simulink model "MultirotorSimPx4HorThrust"  (R2020b)
settings: Solver=VariableStepAuto  StartTime=0.0  StopTime=Simulation.T_END  MaxStep=Simulation.TS_MAX  RelTol=1e-3  EnableMultiTasking=on
PreLoadFcn:
  | % InitializeParameters;
undefined symbols (not defined in the file): Initial, Simulation, Uav
libraries: QuaternionLibrary x26, Px4Library x7, simulink_extras x3
(part 1 of 2)
settings Model: PauseTimes=30  Creator=jban039  LastModifiedBy=jban039
settings DataIOCC: Decimation=10  InitialState=getstatestruct(op)  SaveFormat=StructureWithTime  OutputTimes=Simulation.T_OUT
settings OptimizationCC: LifeSpan=inf
settings DebuggingCC: ReadBeforeWriteMsg=DisableAll  WriteAfterWriteMsg=DisableAll  WriteAfterReadMsg=DisableAll  MultiTaskDSMMsg=none  UnconnectedLineMsg=none  AllowSymbolicDim=off  SFUnexpectedBacktrackingDiag=warning  SFNoUnconditionalDefaultTransitionDiag=warning  SFExecutionAtInitializationDiag=none  ArithmeticOperatorsInVariantConditions=warning
settings ModelReferenceCC: UpdateModelReferenceTargets=IfOutOfDate  ModelReferenceMinAlgLoopOccurrences=on  PropagateSignalLabelsOutOfModel=off
settings SFSimCC: SFSimEcho=off  SimUseLocalCustomCode=off  CustomCodeUndefinedFunction=UseInterfaceOnly
settings RTWCC: RTWUseLocalCustomCode=off
settings CodeAppCC: StateflowObjectComments=on
settings GRTTargetCC: TargetLangStandard=C89/C90 (ANSI)
settings ConfigComp: CovMetricSettings=dw  CovSaveCumulativeToWorkspaceVar=on  CovSaveSingleToWorkspaceVar=on  CovExternalEMLEnable=off

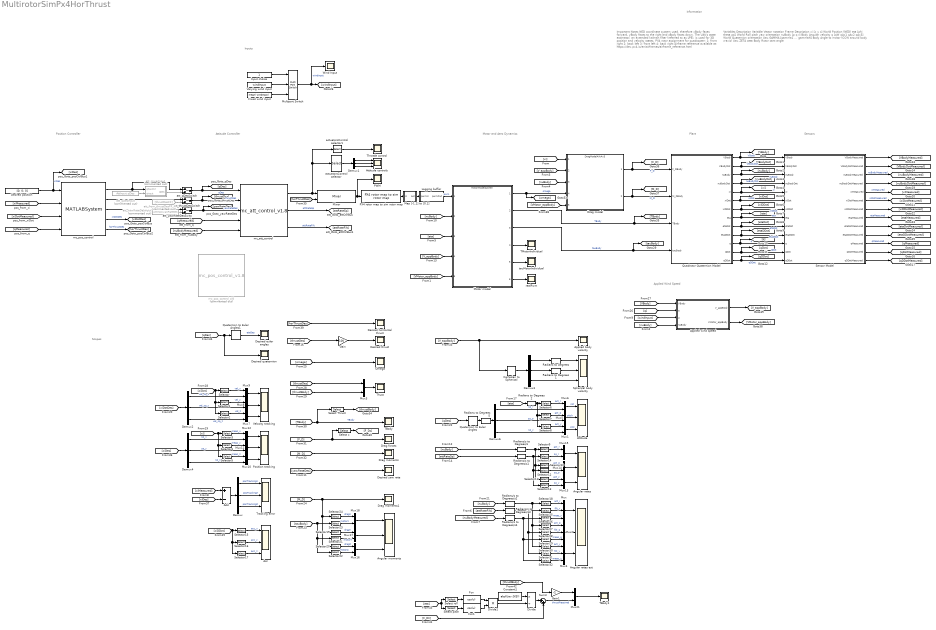
== system MultirotorSimPx4HorThrust ==
  note: Important Notes
      |
      | NED coordinate system used, therefore xBody faces forward, yBody faces to the right and zBody faces down.
      | The UAV's state estimator, an extended kalman filter (referred to as LPE), is used for 3D position and velocity states.
      | PX4 rotor assignment for quadcopter:
      | 1: front right
      | 2: back left
      | 3: front left
      | 4: back right
      | Airframe reference available at:
      | https://dev.px4.io/en/airframes/airframe_reference.html
  note: Applied Wind Speed
  note: Inputs
  note: Scopes
  note: Information
  note: Plant
  note: Motor and Aero Dynamics
  note: Sensors
  note: Attitude Controller
  note: Position Controller
  note: Variables Description
      |
      | Variable
      | Vector notation
      | Frame
      | Description
      |
      | xi
      | [x y z]
      | World
      | Position (NED)
      |
      | eta
      | [phi theta psi]
      | World
      | Roll pitch yaw orientation
      |
      | nuBody
      | [p q r]
      | Body
      | Angular velocity
      |
      | q
      | [qW qAx1 qAx2 qAx3]
      | World
      | Quaternion orientation
      |
      | Uav.GAMMA
      | [gamma1 ... gammaN]
      | Body
      | Angle to motor (CCW around body z-axis)
      |
      | Uav.ZETA
      | zeta
      | Body
      | Rotor cant angle
  Acc : Scope  NumInputPorts=3
  Add : Sum  Inputs=+-
  Angular moments : Scope  NumInputPorts=3
  Angular rates : Scope  NumInputPorts=3
  Angular rates est : Scope  NumInputPorts=3
  Applied body velocity : Scope
  Applied wind speed : Subsystem
  Attitude : Scope  NumInputPorts=3
  Attitude controls : Scope  NumInputPorts=3
  Cartesian to Spherical : QuaternionLibrary/Cartesian to Spherical
  Constant1 : Constant  Value=abs(Uav.G(3))
  Demux{,1..4,6} (6 alike) : Demux  Outputs=3
  Desired euler angles : Scope
  Desired horizontal thrust : Scope
  Desired quaternion : Scope
  Desired thrust : Scope
  Desired position : Constant  Value=[0; 0; 0]
  Desired yaw rate : Scope
  Divide : Product  Inputs=*/
  Divide1 : Product  Inputs=**
  Drag forces : Scope
  Drag model : ModelReference  ModelNameDialog=DragModelAIAAv3  SimulationMode=Normal  ModelReferenceVersion=5.2
  Drag moments : Scope
  Drag moments1 : Scope
  Fcn : Fcn  Expr=cos(u)
  Fcn1 : Fcn  Expr=cos(u)
  Fixed wind input : Constant  Value=mean( windInput )
  Gain : Gain  Gain=100
  Gain1 : Gain  Gain=-1
  Input choice : Constant
  Logging buffer : Subsystem
  Map [-1,1] to [0,1] : Subsystem
  Mixer : Px4Library/Mixer  airframeConfig=5  useHorThrust=1  outputSatStatus=0  SimulateUsing=Code generation
  Motor model : ModelReference  ModelNameDialog=MotorModelZJChen  SimulationMode=Normal  ModelReferenceVersion=5.15
  Multiport Switch : MultiPortSwitch  Inputs=2
  Mux : Mux  Inputs=3
  Mux{1,3,5..18,21} (17 alike) : Mux  Inputs=2
  Mux2 : Mux  Inputs=3
  Mux4 : Mux  Inputs=3
  Omega : Scope
  PWM : Scope
  PX4 rotor map to sim rotor map : Px4Library/PX4 rotor map to sim rotor map  airframeConfig=5  SimulateUsing=Code generation
  Position tracking : Scope  NumInputPorts=3
  Quadrotor Quaternion Model : Subsystem
  Quaternion to Euler Angles : QuaternionLibrary/Quaternion to Euler Angles
  Quaternion to Euler Angles1 : QuaternionLibrary/Quaternion to Euler Angles
  Radians to Degrees {,1..2,5} (4 alike) : QuaternionLibrary/Radians to Degrees   SystemSampleTime=-1  VariantActivationTime=update diagram  Latency=0  AutoFrameSizeCalculation=off
  Radians/s to Degrees/s{,1..4} (5 alike) : QuaternionLibrary/Radians//s to Degrees//s  SystemSampleTime=-1  VariantActivationTime=update diagram  Latency=0  AutoFrameSizeCalculation=off
  Select Thrust : Selector  InputPortWidth=3  IndexOptions=Index vector (dialog)  Indices=[3]  OutputSizes=1
  Select pitch : Selector  InputPortWidth=3  IndexOptions=Index vector (dialog)  Indices=2  OutputSizes=1
  Select roll : Selector  InputPortWidth=3  IndexOptions=Index vector (dialog)  Indices=1  OutputSizes=1
  Select z : Selector  InputPortWidth=3  IndexOptions=Index vector (dialog)  Indices=[3]  OutputSizes=1
  Selector{,3,6,9,14..15,18,23..26} (11 alike) : Selector  InputPortWidth=3  IndexOptions=Index vector (dialog)  Indices=1  OutputSizes=1
  Selector{1,4,7,10,12,16,19,21,27..29} (11 alike) : Selector  InputPortWidth=3  IndexOptions=Index vector (dialog)  Indices=2  OutputSizes=1
  Selector{2,5,8,11,13,17,20,22,30..32} (11 alike) : Selector  InputPortWidth=3  IndexOptions=Index vector (dialog)  Indices=3  OutputSizes=1
  Sensor Model : Subsystem
  Spherical body velocity : Scope  NumInputPorts=3
  Sum3 : Sum  Inputs=|++
  TBody : Scope
  TBody1 : Scope
  TMotorIndividual : Scope
  Throttle control : Scope
  Thust : Scope
  Tracking error : Scope  NumInputPorts=3
  Varying wind input : FromWorkspace  VariableName=windInput
  Velocity tracking : Scope  NumInputPorts=3
  Wind Input : Scope
  actuatorsControl selector : Selector  InputPortWidth=8  IndexOptions=Index vector (dialog)  Indices=[1 2 3]  OutputSizes=1
  actuatorsControl selector1 : Selector  InputPortWidth=8  IndexOptions=Index vector (dialog)  Indices=4  OutputSizes=1
  att_from_thrustDesFF_ff : From  Commented=on  GotoTag=thrustDesFF
  att_mixerInput : Subsystem  Commented=on
  att_qDesInput : FromWorkspace  Commented=on  VariableName=AttInput.qDes  Interpolate=off  OutputAfterFinalValue=Holding final value
  att_qDesSwitch : ManualSwitch
  att_thrustDesSwitch : ManualSwitch
  att_yawRateDesInput : FromWorkspace  Commented=on  VariableName=AttInput.yawRateDes  Interpolate=off  OutputAfterFinalValue=Holding final value
  att_yawRateDesSwitch : ManualSwitch
  mc_att_control : Px4Library/mc_att_control_v1.8  acro_expo_rp=0.69  acro_expo_y=0.69  acro_pitch_max=720  acro_roll_max=720  acro_superexpo_rp=0.7  acro_superexpo_y=0.7  acro_yaw_max=540  airmode=0  d_term_cutoff_freq=30  pitch_rate_d=0.003  pitch_rate_ff=0  pitch_rate_i=0.05  pitch_rate_max=220  pitch_rate_p=0.15  pitch_p=6.5  pitch_rate_integ_lim=0.3  rattitude_thres=0.8  roll_rate_d=0.003  roll_rate_ff=0  roll_rate_i=0.05  roll_rate_max=220  roll_rate_p=0.15  roll_p=6.5  roll_rate_integ_lim=0.3  tpa_breakpoint_d=1  tpa_breakpoint_i=1  tpa_breakpoint_p=1  tpa_rate_d=0  tpa_rate_i=0  tpa_rate_p=0  yaw_rate_d=0  yaw_rate_ff=0  yaw_rate_i=0.1  yaw_rate_max=200  yaw_rate_p=0.2  yaw_auto_max=45  yaw_p=2.8  yaw_rate_integ_lim=0.3  man_throttle_min=0.08  man_tilt_max_deg=35  yaw_rate_scaling=200  throttle_hover=0.5370  throttle_max=1  board_rotation_param=0  board_offset_x=0  board_offset_y=0  board_offset_z=0  bat_scale_en=0  throttle_curve=0  vehicle_status_is_rotary_wing=1  vehicle_status_is_vtol=0  loop_update_rate_hz=250  simple_mode=1  output_rates=1  SimulateUsing=Code generation
  mc_pos_control : MATLABSystem  System=MulticopterPositionControlHorizontal  global_yaw_max_deg=200  mc_att_yaw_p=2.8  mis_yaw_error=12  acceleration_z_max_down=10  acceleration_hor=5  acc_max_estimator_xy=0.5  acceleration_hor_max=10  acceleration_z_max_up=10  alt_mode=0  cruise_speed_90=3  deceleration_hor_slow=5  test_flight_tasks=0  hold_dz=0.1  hold_max_xy=0.8  hold_max_z=0.6  jerk_hor_max=0  jerk_hor_min=1  slow_land_alt1=10  slow_land_alt2=5  land_speed=0.7  manual_thr_max=1  manual_thr_min=0.08  man_tilt_max_deg=35  man_yaw_max_deg=200  thr_hover=0.5  thr_max=1  thr_min=0.12  tilt_max_air_deg=45  tilt_max_land_deg=12  takeoff_ramp_time=0.4  tko_speed=1.5  veld_lp=5  velocity_hor_manual=10  vel_cruise_xy=5  xy_vel_man_expo=0  xy_p=0.95  xy_vel_d=0.01  xy_vel_i=0.02  vel_max_xy_param=12  xy_vel_p=0.09  z_vel_man_expo=0  z_p=1  z_vel_d=0  z_vel_i=0.02  vel_max_down=1  vel_max_up=3  z_vel_p=0.2  nav_rad=10  rc_flt_cutoff=10  rc_flt_smp_rate=50  loop_update_rate_hz=50  simple_mode=1  start_landed=0  ref_lat_init=-36.8509  ref_lon_init=174.7645  ref_alt_init=19  use_hor_thrust=1  controller=Ctrl  controller_op=thrustOp  SimulateUsing=Code generation
      mask Type: MulticopterPositionControlHorizontal
      mask Display:
      | disp(['mc_pos_control' char(10) '' char(10) 'v1.82' char(10) '' char(10) 'HORIZONTAL']);
      | port_label('input',1,'xiDes');
      | port_label('input',2,'xiMeas');
      | port_label('input',3,'xiDotMeas');
      | port_label('input',4,'qMeas');
      | port_label('output',1,'qDes');
      | port_label('output',2,'thrustDes');
      | port_label('output',3,'yawRateDes');
      | port_label('output',4,'xiDotDes');
      | port_label('output',5,'horThrustDes');
  mc_pos_control_old : Px4Library/mc_pos_control_v1.8  Commented=on  global_yaw_max_deg=200  mc_att_yaw_p=2.8  mis_yaw_error=12  acceleration_z_max_down=10  acceleration_hor=5  acc_max_estimator_xy=0.5  acceleration_hor_max=10  acceleration_z_max_up=10  alt_mode=0  cruise_speed_90=3  deceleration_hor_slow=5  test_flight_tasks=0  hold_dz=0.1  hold_max_xy=0.8  hold_max_z=0.6  jerk_hor_max=0  jerk_hor_min=1  slow_land_alt1=1  slow_land_alt2=0.5  land_speed=0.6  manual_thr_max=1  manual_thr_min=0.08  man_tilt_max_deg=35  man_yaw_max_deg=200  thr_hover=0.5370  thr_max=1  thr_min=0.12  tilt_max_air_deg=45  tilt_max_land_deg=12  takeoff_ramp_time=0.4  tko_speed=1.5  veld_lp=5  velocity_hor_manual=10  vel_cruise_xy=5  xy_vel_man_expo=0  xy_p=0.95  xy_vel_d=0.01  xy_vel_i=0.02  vel_max_xy_param=12  xy_vel_p=0.09  z_vel_man_expo=0  z_p=1  z_vel_d=0  z_vel_i=0.02  vel_max_down=1  vel_max_up=3  z_vel_p=0.2  nav_rad=2  rc_flt_cutoff=10  rc_flt_smp_rate=50  loop_update_rate_hz=50  simple_mode=1  start_landed=0  ref_lat_init=-36.8509  ref_lon_init=174.7645  ref_alt_init=19  SimulateUsing=Code generation
  realPwm : Scope
  tauMotorIndividual : Scope
  wires:
  Motor model/1 -> [omega], Drag model/4  "omega"
  Motor model/2 -> Quadrotor Quaternion Model/3(TBody), [TBody]  "TBody"
  Drag model/2 -> Quadrotor Quaternion Model/2(M_DBody), [M_D]  "M_D"
  Quadrotor Quaternion Model/1(VBody) -> Sensor Model/1(VBody), [VBody]  "VBody"
  Quadrotor Quaternion Model/2(VBodyDot) -> Sensor Model/2(VBodyDot), [VBodyDot]  "VBodyDot"
  Quadrotor Quaternion Model/3(nuBody) -> Sensor Model/3(nuBody), [nuBody]  "nuBody"
  Quadrotor Quaternion Model/4(nuBodyDot) -> Sensor Model/4(nuBodyDot), [nuBodyDot]  "nuBodyDot"
  Quadrotor Quaternion Model/5(xi) -> Sensor Model/5(xi), [xi]  "xi"
  Quadrotor Quaternion Model/6(xiDot) -> Sensor Model/6(xiDot), [xiDot]  "xiDot"
  Quadrotor Quaternion Model/7(xiDDot) -> Sensor Model/7(xiDDot), [xiDDot]  "xiDDot"
  Quadrotor Quaternion Model/8(eta) -> Sensor Model/8(eta), [eta]  "eta"
  Quadrotor Quaternion Model/9(etaDot) -> Sensor Model/9(etaDot), [etaDot]  "etaDot"
  Quadrotor Quaternion Model/10(etaDDot) -> Sensor Model/10(etaDDot), [etaDDot]  "etaDDot"
  [V_appBody] -> Drag model/2
  [nuBody] -> Motor model/2
  Quadrotor Quaternion Model/11(q) -> Sensor Model/11(q), [q]  "q"
  Quadrotor Quaternion Model/12(qDot) -> Sensor Model/12(qDot), [qDot]  "qDot"
  Quadrotor Quaternion Model/13(qDDot) -> Sensor Model/13(qDDot), [qDDot]  "qDDot"
  Drag model/1 -> Quadrotor Quaternion Model/1(F_DBody), [F_D]  "F_D"
  Sensor Model/1(VBodyMeasured) -> [VBodyMeasured]
  Sensor Model/2(VBodyDotMeasured) -> [VBodyDotMeasured]
  Sensor Model/3(nuBodyMeasured) -> [nuBodyMeasured]  "nuBodyMeasured"
  Sensor Model/4(nuBodyDotMeasured) -> [nuBodyDotMeasured]
  Sensor Model/5(xiMeasured) -> [xiMeasured]  "xiMeasured"
  Sensor Model/6(xiDotMeasured) -> [xiDotMeasured]  "xiDotMeasured"
  Sensor Model/7(xiDDotMeasured) -> [xiDDotMeasured]
  Sensor Model/8(etaMeasured) -> [etaMeasured]  "etaMeasured"
  Sensor Model/9(etaDotMeasured) -> [etaDotMeasured]
  Sensor Model/10(etaDDotMeasured) -> [etaDDotMeasured]
  Sensor Model/11(qMeasured) -> [qMeasured]  "qMeasured"
  Sensor Model/12(qDotMeasured) -> [qDotMeasured]
  Sensor Model/13(qDDotMeasured) -> [qDDotMeasured]
  Logging buffer/1(pwmOut) -> Motor model/1  "pwm"
  [qMeasured] -> mc_att_control/4
  [nuBodyMeasured] -> mc_att_control/5
  [qMeasured] -> mc_pos_control/4
  mc_pos_control/3 -> att_yawRateDesSwitch/1
  [xiDotMeasured] -> mc_pos_control/3
  [xiMeasured] -> mc_pos_control/2
  Selector6/1 -> Mux6/1  "act_r"
  Selector7/1 -> Mux5/1  "act_p"
  Mux7/1 -> Velocity tracking/3
  Mux8/1 -> Velocity tracking/2
  Mux9/1 -> Velocity tracking/1
  Demux2/1 -> Mux9/2  "vel_sp_x"
  Selector/1 -> Mux9/1  "vel_x"
  Demux2/2 -> Mux8/2  "vel_sp_y"
  Selector1/1 -> Mux8/1  "vel_y"
  Demux2/3 -> Mux7/2  "vel_sp_z"
  Selector2/1 -> Mux7/1  "vel_z"
  Mux10/1 -> Position tracking/3
  Mux11/1 -> Position tracking/2
  Mux12/1 -> Position tracking/1
  Demux4/1 -> Mux12/2  "sp_x"
  Selector3/1 -> Mux12/1  "meas_x"
  Demux4/2 -> Mux11/2  "sp_y"
  Selector4/1 -> Mux11/1  "meas_y"
  Demux4/3 -> Mux10/2  "sp_z"
  Selector5/1 -> Mux10/1  "meas_z"
  Quaternion to Euler Angles/1 -> Radians to Degrees 5/1
  Demux6/1 -> Mux6/2  "sp_r"
  Demux6/2 -> Mux5/2  "sp_p"
  Demux6/3 -> Mux1/2  "sp_y"
  Selector8/1 -> Mux1/1  "act_y"
  [qDes] -> Quaternion to Euler Angles/1
  Mixer/1 -> PX4 rotor map to sim rotor map/1, PWM/1
  Map [-1,1] to [0,1]/1(out) -> Logging buffer/1(pwmIn)
  Add/1 -> Demux/1
  Demux/1 -> Tracking error/1  "posTrackingX"
  Demux/2 -> Tracking error/2  "posTrackingY"
  Demux/3 -> Tracking error/3  "posTrackingZ"
  [nuBody] -> Drag model/3
  Mux6/1 -> Attitude/1  "roll"
  Mux5/1 -> Attitude/2  "pitch"
  [eta] -> Motor model/3
  [xiDot] -> Selector2/1, Selector1/1, Selector/1
  [xi] -> Selector5/1, Selector4/1, Selector3/1
  [xiMeasured] -> Add/1
  Multiport Switch/1 -> Wind Input/1, [windInput]  "windInput"
  [V_appBody] -> Motor model/4
  mc_pos_control/4 -> [xiDotDes]  "xiDotDes"
  mc_att_control/2 -> [attRateSp]  "attRateSp"
  [omega] -> Omega/1
  Radians to Degrees 5/1 -> Demux6/1
  Radians to Degrees 2/1 -> Selector8/1, Selector7/1, Selector6/1
  [eta] -> Radians to Degrees 2/1
  Motor model/4 -> TMotorIndividual/1
  [thrustDes] -> Mux3/1
  [thrustBody] -> Mux3/2
  Mux3/1 -> Thust/1
  Motor model/5 -> tauMotorIndividual/1
  [xi] -> Drag model/1
  [TBody] -> Select Thrust/1, TBody/1  "TBody"
  Select Thrust/1 -> [thrustBody]
  [F_D] -> Drag forces/1, Select z/1
  [V_appBody] -> Cartesian to Spherical/1, Applied body velocity/1
  Demux3/1 -> "Radians to Degrees "/1
  Demux3/2 -> Radians to Degrees 1/1
  Demux3/3 -> Spherical body velocity/3
  "Radians to Degrees "/1 -> Spherical body velocity/1
  Radians to Degrees 1/1 -> Spherical body velocity/2
  [M_D] -> Drag moments/1
  [VMotor_appBody] -> Motor model/5
  [VMotor_appBody] -> Drag model/5
  att_qDesSwitch/1 -> mc_att_control/1, [qDes]  "qDes"
  att_thrustDesSwitch/1 -> mc_att_control/2, [thrustDes]  "thrustDes"
  att_yawRateDesSwitch/1 -> mc_att_control/3, [yawRateDes]  "yawRateDes"
  att_yawRateDesInput/1 -> att_yawRateDesSwitch/2
  att_from_thrustDesFF_ff/1 -> att_thrustDesSwitch/2
  [yawRateDes] -> Desired yaw rate/1
  Mux1/1 -> Attitude/3  "yaw"
  Motor model/3 -> Quadrotor Quaternion Model/4(tauBody), [tauBody]  "tauBody"
  [VBody] -> Applied wind speed/1(VBody)
  [q] -> Applied wind speed/2(q)
  [windInput] -> Applied wind speed/3(U)
  Applied wind speed/1(V_appBody) -> [V_appBody]
  Applied wind speed/2(VMotor_appBody) -> [VMotor_appBody]
  [nuBody] -> Applied wind speed/4(nuBody)
  Selector9/1 -> Mux15/1  "act_r"
  Selector10/1 -> Mux14/1  "act_p"
  Selector11/1 -> Mux13/1  "act_y"
  Mux15/1 -> Angular rates/1
  Mux14/1 -> Angular rates/2
  Radians/s to Degrees/s/1 -> Selector9/1, Selector11/1, Selector10/1
  [nuBody] -> Radians/s to Degrees/s/1
  Mux13/1 -> Angular rates/3
  Radians/s to Degrees/s1/1 -> Selector14/1, Selector13/1, Selector12/1
  Selector14/1 -> Mux15/2  "sp_r"
  Selector12/1 -> Mux14/2  "sp_p"
  Selector13/1 -> Mux13/2  "sp_y"
  [attRateSp] -> Radians/s to Degrees/s1/1
  Selector15/1 -> Acc/1  "acc_x"
  Selector16/1 -> Acc/2  "acc_y"
  Selector17/1 -> Acc/3  "acc_z"
  [xiDDot] -> Selector15/1, Selector16/1, Selector17/1
  [thrustDes] -> Gain/1
  actuatorsControl selector/1 -> Demux1/1
  [M_D] -> Selector20/1, Selector19/1, Selector24/1, Drag moments1/1
  Mux18/1 -> Angular moments/1
  Mux17/1 -> Angular moments/2
  Mux16/1 -> Angular moments/3
  Selector24/1 -> Mux18/1  "dragX"
  Selector23/1 -> Mux18/2  "motorX"
  Selector19/1 -> Mux17/1  "dragY"
  Selector21/1 -> Mux17/2  "motorY"
  Selector20/1 -> Mux16/1  "dragZ"
  Selector22/1 -> Mux16/2  "MotorZ"
  [tauBody] -> Selector22/1, Selector21/1, Selector23/1
  Desired position/1 -> [xiDes], mc_pos_control/1  "xiDes"
  [qDes] -> Desired quaternion/1, Quaternion to Euler Angles1/1
  Quaternion to Euler Angles1/1 -> Desired euler angles/1  "etaDes"
  Divide/1 -> Sum3/1
  Sum3/1 -> Mux21/2  "thrustRequired"
  Mux21/1 -> TBody1/1
  Constant1/1 -> Divide/1
  Select z/1 -> [F_Dz]
  [thrustBody] -> Gain1/1
  [eta] -> Select pitch/1, Select roll/1
  Select roll/1 -> Fcn/1
  Select pitch/1 -> Fcn1/1
  Fcn/1 -> Divide1/1
  Fcn1/1 -> Divide1/2
  Divide1/1 -> Divide/2
  [F_Dz] -> Sum3/2
  mc_pos_control/1 -> att_qDesSwitch/1, att_mixerInput/1(qPosCtrl)
  mc_pos_control/2 -> att_thrustDesSwitch/1
  att_mixerInput/1(qDes) -> att_qDesSwitch/2
  att_qDesInput/1 -> att_mixerInput/2(qInput)
  Motor model/6 -> realPwm/1
  Cartesian to Spherical/1 -> Demux3/1
  mc_att_control/1 -> actuatorsControl selector1/1, actuatorsControl selector/1, Mixer/1
  Input choice/1 -> Multiport Switch/1
  Fixed wind input/1 -> Multiport Switch/3
  Varying wind input/1 -> Multiport Switch/2
  [xiDotDes] -> Demux2/1
  [xiDes] -> Demux4/1
  [xiDes] -> Add/2
  Gain/1 -> Desired thrust/1
  mc_att_control/3 -> [attRateFilt]  "attRateFilt"
  [nuBody] -> Radians/s to Degrees/s2/1
  [attRateFilt] -> Radians/s to Degrees/s3/1
  [nuBodyMeasured] -> Radians/s to Degrees/s4/1
  Radians/s to Degrees/s2/1 -> Selector30/1, Selector27/1, Selector18/1
  Radians/s to Degrees/s3/1 -> Selector31/1, Selector28/1, Selector25/1
  Radians/s to Degrees/s4/1 -> Selector29/1, Selector32/1, Selector26/1
  Selector25/1 -> Mux/2  "filt_r"
  Selector18/1 -> Mux/1  "act_r"
  Selector26/1 -> Mux/3  "meas_r"
  Selector29/1 -> Mux2/3  "meas_p"
  Selector27/1 -> Mux2/1  "act_p"
  Selector28/1 -> Mux2/2  "filt_p"
  Selector30/1 -> Mux4/1  "act_y"
  Selector31/1 -> Mux4/2  "filt_y"
  Selector32/1 -> Mux4/3  "meas_y"
  Mux2/1 -> Angular rates est/2
  Mux/1 -> Angular rates est/1
  Mux4/1 -> Angular rates est/3
  actuatorsControl selector1/1 -> Throttle control/1
  PX4 rotor map to sim rotor map/1 -> Map [-1,1] to [0,1]/1(in)
  Demux1/1 -> Attitude controls/1
  Demux1/2 -> Attitude controls/2
  Demux1/3 -> Attitude controls/3
  Gain1/1 -> Mux21/1
  mc_pos_control/5 -> [horThrustDes]  "horThrustDes"
  [horThrustDes] -> Mixer/2
  [horThrustDes] -> Desired horizontal thrust/1

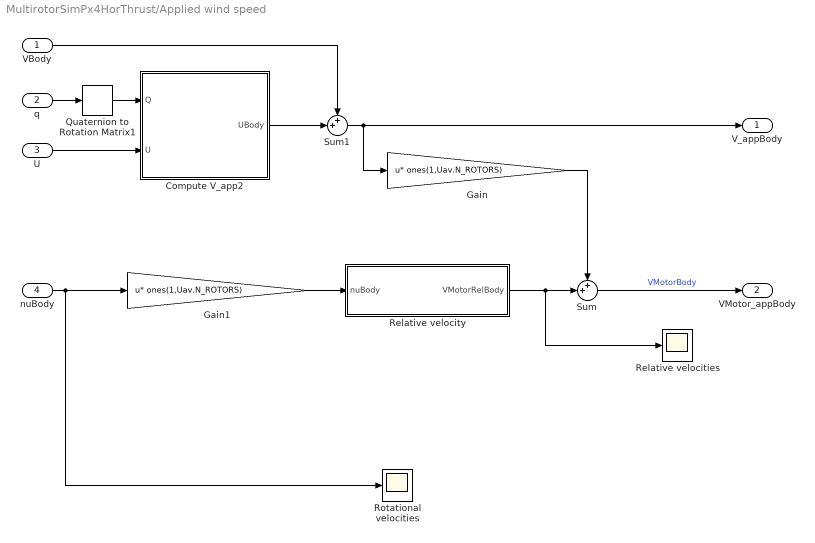
== system MultirotorSimPx4HorThrust/Applied wind speed ==
  VBody : Inport  Unit=m/s
  q : Inport  Port=2
  U : Inport  Port=3  Unit=m/s
  nuBody : Inport  Port=4  Unit=rad/s
  Compute V_app2 : MATLAB Function  TreatAsAtomicUnit=on
  Gain : Gain  Gain=ones(1,Uav.N_ROTORS)  Multiplication=Matrix(u*K)
  Gain1 : Gain  Gain=ones(1,Uav.N_ROTORS)  Multiplication=Matrix(u*K)
  Quaternion to Rotation Matrix1 : QuaternionLibrary/Quaternion to Rotation Matrix
  Relative velocities : Scope
  Relative velocity : MATLAB Function  TreatAsAtomicUnit=on
  Rotational velocities : Scope
  Sum : Sum  Inputs=++|
  Sum1 : Sum  Inputs=++|
  V_appBody : Outport  Unit=m/s  VectorParamsAs1DForOutWhenUnconnected=off
  VMotor_appBody : Outport  Port=2  Unit=m/s  PortDimensions=[3,Uav.N_ROTORS]  VectorParamsAs1DForOutWhenUnconnected=off
  wires:
  U/1 -> Compute V_app2/2(U)
  Sum/1 -> VMotor_appBody/1  "VMotorBody"
  Quaternion to Rotation Matrix1/1 -> Compute V_app2/1(Q)
  nuBody/1 -> Gain1/1, Rotational velocities/1
  Gain/1 -> Sum/1
  VBody/1 -> Sum1/1
  q/1 -> Quaternion to Rotation Matrix1/1
  Relative velocity/1(VMotorRelBody) -> Relative velocities/1, Sum/2
  Compute V_app2/1(UBody) -> Sum1/2
  Sum1/1 -> Gain/1, V_appBody/1
  Gain1/1 -> Relative velocity/1(nuBody)

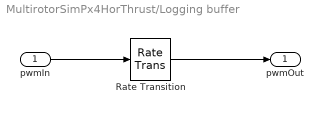
== system MultirotorSimPx4HorThrust/Logging buffer ==
  pwmIn : Inport
  Rate Transition : RateTransition
  pwmOut : Outport  VectorParamsAs1DForOutWhenUnconnected=off
  wires:
  pwmIn/1 -> Rate Transition/1
  Rate Transition/1 -> pwmOut/1

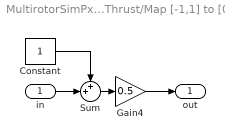
== system MultirotorSimPx4HorThrust/Map [-1,1] to [0,1] ==
  in : Inport
  Constant : Constant
  Gain4 : Gain  Gain=0.5
  Sum : Sum  Inputs=++|
  out : Outport  VectorParamsAs1DForOutWhenUnconnected=off
  wires:
  Constant/1 -> Sum/1
  in/1 -> Sum/2
  Gain4/1 -> out/1
  Sum/1 -> Gain4/1

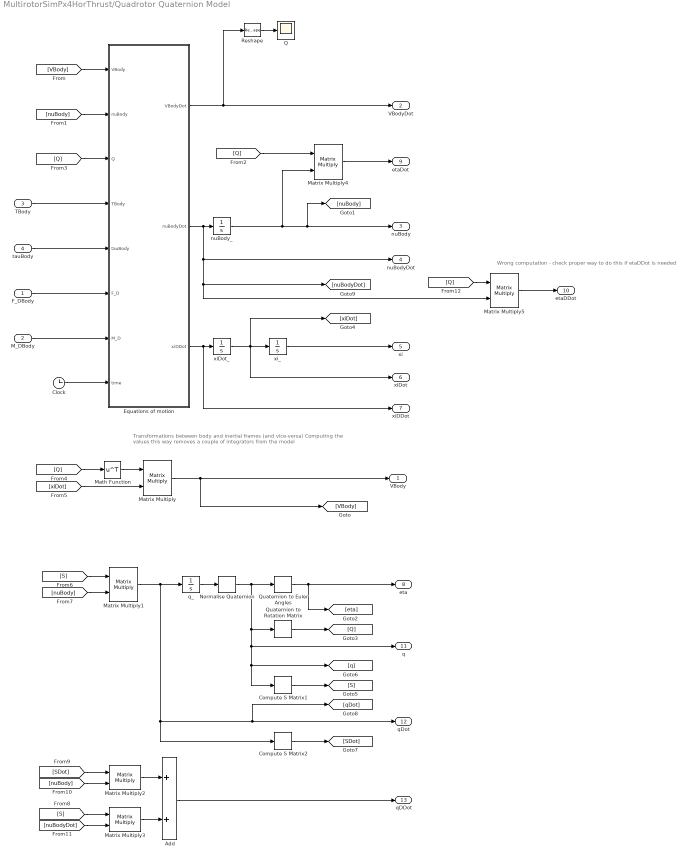
== system MultirotorSimPx4HorThrust/Quadrotor Quaternion Model ==
  note: Wrong computation - check proper way to do this if etaDDot is needed
  note: Transformations between body and inertial frames (and vice-versa)
      | Computing the values this way removes a couple of integrators from the model
  F_DBody : Inport  Unit=N
  M_DBody : Inport  Port=2  Unit=N*m
  TBody : Inport  Port=3  Unit=N
  tauBody : Inport  Port=4  Unit=N*m
  Add : Sum
  Clock : Clock
  Compute S Matrix1 : QuaternionLibrary/Compute S Matrix
  Compute S Matrix2 : QuaternionLibrary/Compute S Matrix
  Equations of motion : MATLAB Function  TreatAsAtomicUnit=on
  Math Function : Math  Operator=transpose  SignedPower=on  SaturateOnIntegerOverflow=on
  Matrix Multiply{,1..5} (6 alike) : Product  Multiplication=Matrix(*)
  Normalise Quaternion : QuaternionLibrary/Normalise Quaternion
  Q : Scope
  Quaternion to Euler Angles : QuaternionLibrary/Quaternion to Euler Angles
  Quaternion to Rotation Matrix : QuaternionLibrary/Quaternion to Rotation Matrix
  Reshape : Reshape  OutputDimensionality=Column vector (2-D)
  nuBody_ : Integrator  InitialCondition=Initial.NU_BODY  ContinuousStateAttributes='nuBody'
  q_ : Integrator  InitialCondition=Initial.Q  ContinuousStateAttributes='q'
  xiDot_ : Integrator  InitialCondition=Initial.XI_DOT  ContinuousStateAttributes='xiDot'
  xi_ : Integrator  InitialCondition=Initial.XI  ContinuousStateAttributes='xi'
  VBody : Outport  Unit=m/s  VectorParamsAs1DForOutWhenUnconnected=off
  VBodyDot : Outport  Port=2  Unit=m/s^2  VectorParamsAs1DForOutWhenUnconnected=off
  nuBody : Outport  Port=3  Unit=rad/s  VectorParamsAs1DForOutWhenUnconnected=off
  nuBodyDot : Outport  Port=4  Unit=rad/s^2  VectorParamsAs1DForOutWhenUnconnected=off
  xi : Outport  Port=5  Unit=m  VectorParamsAs1DForOutWhenUnconnected=off
  xiDot : Outport  Port=6  Unit=m/s  VectorParamsAs1DForOutWhenUnconnected=off
  xiDDot : Outport  Port=7  Unit=m/s^2  VectorParamsAs1DForOutWhenUnconnected=off
  eta : Outport  Port=8  Unit=rad  VectorParamsAs1DForOutWhenUnconnected=off
  etaDot : Outport  Port=9  Unit=rad/s  VectorParamsAs1DForOutWhenUnconnected=off
  etaDDot : Outport  Port=10  Unit=rad/s^2  VectorParamsAs1DForOutWhenUnconnected=off
  q : Outport  Port=11  VectorParamsAs1DForOutWhenUnconnected=off
  qDot : Outport  Port=12  VectorParamsAs1DForOutWhenUnconnected=off
  qDDot : Outport  Port=13  VectorParamsAs1DForOutWhenUnconnected=off
  wires:
  Equations of motion/1(VBodyDot) -> Reshape/1, VBodyDot/1
  xi_/1 -> xi/1
  [nuBody] -> Equations of motion/2(nuBody)
  [VBody] -> Equations of motion/1(VBody)
  tauBody/1 -> Equations of motion/5(tauBody)
  TBody/1 -> Equations of motion/4(TBody)
  Equations of motion/3(xiDDot) -> xiDot_/1, xiDDot/1
  F_DBody/1 -> Equations of motion/6(F_D)
  Matrix Multiply/1 -> VBody/1, [VBody]
  M_DBody/1 -> Equations of motion/7(M_D)
  nuBody_/1 -> Matrix Multiply4/2, [nuBody], nuBody/1
  Equations of motion/2(nuBodyDot) -> nuBody_/1, nuBodyDot/1, Matrix Multiply5/2, [nuBodyDot]
  q_/1 -> Normalise Quaternion/1
  Quaternion to Euler Angles/1 -> eta/1, [eta]
  Matrix Multiply4/1 -> etaDot/1
  Quaternion to Rotation Matrix/1 -> [Q]
  [Q] -> Equations of motion/3(Q)
  [Q] -> Math Function/1
  [xiDot] -> Matrix Multiply/2
  Math Function/1 -> Matrix Multiply/1
  [S] -> Matrix Multiply1/1
  [nuBody] -> Matrix Multiply1/2
  Compute S Matrix2/1 -> [SDot]
  [S] -> Matrix Multiply3/1
  Matrix Multiply1/1 -> qDot/1, [qDot], Compute S Matrix2/1, q_/1
  [SDot] -> Matrix Multiply2/1
  [nuBody] -> Matrix Multiply2/2
  [nuBodyDot] -> Matrix Multiply3/2
  Matrix Multiply2/1 -> Add/1
  Matrix Multiply3/1 -> Add/2
  Normalise Quaternion/1 -> Quaternion to Euler Angles/1, q/1, Compute S Matrix1/1, [q], Quaternion to Rotation Matrix/1
  Compute S Matrix1/1 -> [S]
  [Q] -> Matrix Multiply4/1
  Add/1 -> qDDot/1
  [Q] -> Matrix Multiply5/1
  Matrix Multiply5/1 -> etaDDot/1
  Reshape/1 -> Q/1
  xiDot_/1 -> xi_/1, [xiDot], xiDot/1
  Clock/1 -> Equations of motion/8(time)

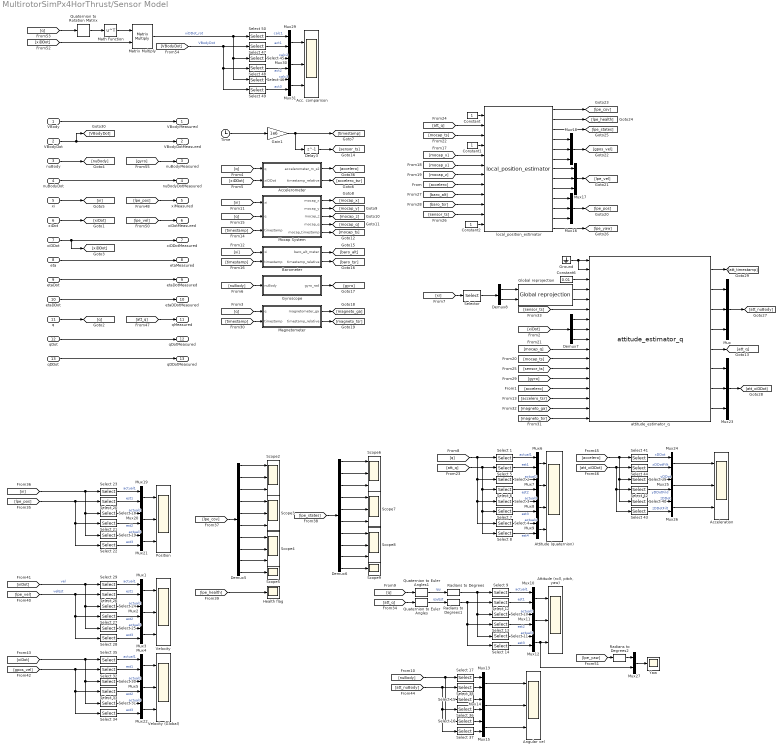
== system MultirotorSimPx4HorThrust/Sensor Model ==
  VBody : Inport  Unit=m/s  PortDimensions=3
  VBodyDot : Inport  Port=2  Unit=m/s^2  PortDimensions=3
  nuBody : Inport  Port=3  Unit=rad/s  PortDimensions=3
  nuBodyDot : Inport  Port=4  Unit=rad/s^2  PortDimensions=3
  xi : Inport  Port=5  Unit=m  PortDimensions=3
  xiDot : Inport  Port=6  Unit=m/s  PortDimensions=3
  xiDDot : Inport  Port=7  Unit=m/s^2  PortDimensions=3
  eta : Inport  Port=8  Unit=rad  PortDimensions=3
  etaDot : Inport  Port=9  Unit=rad/s  PortDimensions=3
  etaDDot : Inport  Port=10  Unit=rad/s^2  PortDimensions=3
  q : Inport  Port=11  PortDimensions=4
  qDot : Inport  Port=12  PortDimensions=4
  qDDot : Inport  Port=13  PortDimensions=4
  Acc. comparison : Scope  NumInputPorts=3
  Acceleration : Scope  NumInputPorts=3
  Accelerometer : Subsystem
  Angular vel : Scope  NumInputPorts=3
  Attitude (quaternion) : Scope  NumInputPorts=4
  "Attitude (roll, pitch, yaw)" : Scope  NumInputPorts=3
  Barometer : Subsystem
  Constant : Constant
  Constant1 : Constant
  Constant2 : Constant
  Constant6 : Constant  Value=0.01
  Delay3 : Delay  DelayLength=1  SampleTime=1/400
  Demux5 : Demux  Outputs=10
  Demux6 : Demux  Outputs=10
  Demux7 : Demux  Outputs=3
  Demux8 : Demux  Outputs=2
  Gain1 : Gain  Gain=1e6
  Global reprojection : Px4Library/Global reprojection  LAT0=-36.865577  LON0=174.772065
  Ground : Ground
  Gyroscope : Subsystem
  Health flag : Scope
  Magnetometer : Subsystem
  Math Function : Math  Operator=transpose  SignedPower=on  SaturateOnIntegerOverflow=on
  Matrix Multiply : Product  Multiplication=Matrix(*)
  Mocap System : Subsystem
  Mux{,16..18,23} (5 alike) : Mux  Inputs=3
  Mux{1..15,19..22,24..27,29..31} (26 alike) : Mux  Inputs=2
  Position : Scope  NumInputPorts=3
  Quaternion to Euler Angles : QuaternionLibrary/Quaternion to Euler Angles
  Quaternion to Euler Angles1 : QuaternionLibrary/Quaternion to Euler Angles
  Quaternion to Rotation Matrix : QuaternionLibrary/Quaternion to Rotation Matrix
  Radians to Degrees : simulink_extras/Transformations/Radians to Degrees
  Radians to Degrees1 : simulink_extras/Transformations/Radians to Degrees
  Radians to Degrees2 : simulink_extras/Transformations/Radians to Degrees
  Scope{2..4,6..8} (6 alike) : Scope  NumInputPorts=3
  Scope5 : Scope
  Scope9 : Scope
  Select 1 : Selector  InputPortWidth=4  IndexOptions=Index vector (dialog)  Indices=1  OutputSizes=1
  Select {10,13,15,18,21,24,27,30,33,36,39,42,45,48} (14 alike) : Selector  InputPortWidth=3  IndexOptions=Index vector (dialog)  Indices=2  OutputSizes=1
  Select {11,14,16,19,22,25,28,31,34,37,40,43,46,49} (14 alike) : Selector  InputPortWidth=3  IndexOptions=Index vector (dialog)  Indices=3  OutputSizes=1
  Select {9,12,17,20,23,26,29,32,35,38,41,44,47,50} (14 alike) : Selector  InputPortWidth=3  IndexOptions=Index vector (dialog)  Indices=1  OutputSizes=1
  Select 2 : Selector  InputPortWidth=4  IndexOptions=Index vector (dialog)  Indices=2  OutputSizes=1
  Select 3 : Selector  InputPortWidth=4  IndexOptions=Index vector (dialog)  Indices=3  OutputSizes=1
  Select 4 : Selector  InputPortWidth=4  IndexOptions=Index vector (dialog)  Indices=4  OutputSizes=1
  Select 5 : Selector  InputPortWidth=4  IndexOptions=Index vector (dialog)  Indices=1  OutputSizes=1
  Select 6 : Selector  InputPortWidth=4  IndexOptions=Index vector (dialog)  Indices=2  OutputSizes=1
  Select 7 : Selector  InputPortWidth=4  IndexOptions=Index vector (dialog)  Indices=3  OutputSizes=1
  Select 8 : Selector  InputPortWidth=4  IndexOptions=Index vector (dialog)  Indices=4  OutputSizes=1
  Selector : Selector  InputPortWidth=3  IndexOptions=Index vector (dialog)  Indices=[1 2]  OutputSizes=1
  Time : Clock
  Velocity : Scope  NumInputPorts=3
  Velocity (Global) : Scope  NumInputPorts=3
  Yaw : Scope
  attitude_estimator_q : Px4Library/attitude_estimator_q  Q_SAMPLING_PERIOD=1/250  INIT_Q=[1 0 0 0]  ATT_W_ACC=0.2  ATT_W_MAG=0.1  ATT_W_EXT_HDG=0.1  ATT_W_GYRO_BIAS=0.1  ATT_MAG_DECL=0.0  ATT_MAG_DECL_A=1  ATT_EXT_HDG_M=2  ATT_ACC_COMP=1  ATT_BIAS_MAX=0.05  FW_ARSP_MODE=0
  local_position_estimator : Px4Library/local_position_estimator  LPE_SAMPLING_PERIOD=0.01  LPE_ACC_XY=0.012  LPE_ACC_Z=0.02  LPE_BAR_Z=3  LPE_EPH_MAX=3  LPE_EPV_MAX=5  LPE_FAKE_ORIGIN=0  LPE_FGYRO_HP=0.001  LPE_FLW_OFF_Z=0  LPE_FLW_QMIN=150  LPE_FLW_R=7  LPE_FLW_RR=7  LPE_FLW_SCALE=1.3  LPE_GPS_DELAY=0.29  LPE_GPS_VXY=0.25  LPE_GPS_VZ=0.25  LPE_GPS_XY=1  LPE_GPS_Z=3  LPE_LAND_VXY=0.05  LPE_LAND_Z=0.03  LPE_LAT=47.3977  LPE_LDR_OFF_Z=0  LPE_LDR_Z=0.03  LPE_LON=8.5456  LPE_PN_B=0.001  LPE_PN_P=0.1  LPE_PN_T=0.001  LPE_PN_V=0.1  LPE_SNR_OFF_Z=0  LPE_SNR_Z=0.05  LPE_T_MAX_GRADE=1  LPE_VIC_P=0.001  LPE_VIS_DELAY=0.1  LPE_VIS_XY=0.1  LPE_VIS_Z=0.5  LPE_VXY_PUB=0.3  LPE_X_LP=5  LPE_Z_PUB=1  LPE_FUSION=193  Barometer=on  GPS=off  LIDAR=off  Flow=off  Sonar=off  Vision=off  Mocap=on  Land=on
  VBodyMeasured : Outport  Unit=m/s  VectorParamsAs1DForOutWhenUnconnected=off
  VBodyDotMeasured : Outport  Port=2  Unit=m/s^2  VectorParamsAs1DForOutWhenUnconnected=off
  nuBodyMeasured : Outport  Port=3  Unit=rad/s  VectorParamsAs1DForOutWhenUnconnected=off
  nuBodyDotMeasured : Outport  Port=4  Unit=rad/s^2  VectorParamsAs1DForOutWhenUnconnected=off
  xiMeasured : Outport  Port=5  Unit=m  VectorParamsAs1DForOutWhenUnconnected=off
  xiDotMeasured : Outport  Port=6  Unit=m/s  VectorParamsAs1DForOutWhenUnconnected=off
  xiDDotMeasured : Outport  Port=7  Unit=m/s^2  VectorParamsAs1DForOutWhenUnconnected=off
  etaMeasured : Outport  Port=8  Unit=rad  VectorParamsAs1DForOutWhenUnconnected=off
  etaDotMeasured : Outport  Port=9  Unit=rad/s  VectorParamsAs1DForOutWhenUnconnected=off
  etaDDotMeasured : Outport  Port=10  Unit=rad/s^2  VectorParamsAs1DForOutWhenUnconnected=off
  qMeasured : Outport  Port=11  VectorParamsAs1DForOutWhenUnconnected=off
  qDotMeasured : Outport  Port=12  VectorParamsAs1DForOutWhenUnconnected=off
  qDDotMeasured : Outport  Port=13  VectorParamsAs1DForOutWhenUnconnected=off
  wires:
  xiDot/1 -> [xiDot]
  xi/1 -> [xi]
  nuBodyDot/1 -> nuBodyDotMeasured/1
  nuBody/1 -> [nuBody]
  VBodyDot/1 -> [VBodyDot], VBodyDotMeasured/1
  VBody/1 -> VBodyMeasured/1
  eta/1 -> etaMeasured/1
  etaDot/1 -> etaDotMeasured/1
  etaDDot/1 -> etaDDotMeasured/1
  q/1 -> [q]
  qDot/1 -> qDotMeasured/1
  qDDot/1 -> qDDotMeasured/1
  [att_q] -> local_position_estimator/2
  [mocap_x] -> local_position_estimator/5
  [mocap_z] -> local_position_estimator/7
  local_position_estimator/10 -> Mux16/1
  local_position_estimator/11 -> Mux16/2
  local_position_estimator/12 -> Mux16/3
  Demux5/2 -> Scope2/2
  Demux5/1 -> Scope2/1
  Demux5/3 -> Scope2/3
  Demux5/4 -> Scope3/1
  Demux5/5 -> Scope3/2
  Demux5/6 -> Scope3/3
  Demux5/7 -> Scope4/1
  Demux5/8 -> Scope4/2
  Demux5/9 -> Scope4/3
  Demux5/10 -> Scope5/1
  [lpe_states] -> Demux6/1
  Demux6/2 -> Scope6/2
  Demux6/1 -> Scope6/1
  Demux6/3 -> Scope6/3
  Demux6/4 -> Scope7/1
  Demux6/5 -> Scope7/2
  Demux6/6 -> Scope7/3
  Demux6/7 -> Scope8/1
  Demux6/8 -> Scope8/2
  Demux6/9 -> Scope8/3
  Demux6/10 -> Scope9/1
  Constant1/1 -> local_position_estimator/4
  [lpe_health] -> Health flag/1
  Constant/1 -> local_position_estimator/1
  [mocap_ts] -> local_position_estimator/3
  [xiDot] -> Demux7/1
  Time/1 -> Gain1/1
  [accelero_tsr] -> attitude_estimator_q/15
  Global reprojection/1 -> attitude_estimator_q/4
  Global reprojection/2 -> attitude_estimator_q/5
  [xi] -> Selector/1
  Selector/1 -> Demux8/1
  Demux8/1 -> Global reprojection/1
  Demux8/2 -> Global reprojection/2
  [att_q] -> Select 8/1, Select 7/1, Select 6/1, Select 5/1
  [q] -> Select 2/1, Select 3/1, Select 4/1, Select 1/1
  Mux6/1 -> Attitude (quaternion)/1
  Mux7/1 -> Attitude (quaternion)/2
  Mux8/1 -> Attitude (quaternion)/3
  Mux9/1 -> Attitude (quaternion)/4
  Select 4/1 -> Mux9/1  "actual4"
  Select 8/1 -> Mux9/2  "est4"
  Select 3/1 -> Mux8/1  "actual3"
  Select 7/1 -> Mux8/2  "est3"
  Select 6/1 -> Mux7/2  "est2"
  Select 2/1 -> Mux7/1  "actual2"
  Select 5/1 -> Mux6/2  "est1"
  Select 1/1 -> Mux6/1  "actual1"
  Constant6/1 -> attitude_estimator_q/3
  [q] -> Magnetometer/1(q)
  Mux10/1 -> "Attitude (roll, pitch, yaw)"/1
  Mux11/1 -> "Attitude (roll, pitch, yaw)"/2
  Mux12/1 -> Mux27/2, "Attitude (roll, pitch, yaw)"/3
  Select 11/1 -> Mux12/1  "actual3"
  Select 14/1 -> Mux12/2  "est3"
  Select 13/1 -> Mux11/2  "est2"
  Select 10/1 -> Mux11/1  "actual2"
  Select 12/1 -> Mux10/2  "est1"
  Select 9/1 -> Mux10/1  "actual1"
  [q] -> Quaternion to Euler Angles1/1
  Quaternion to Euler Angles1/1 -> Radians to Degrees/1  "rpy"
  Quaternion to Euler Angles/1 -> Radians to Degrees1/1  "rpyEst"
  Mux13/1 -> Angular vel/1
  Mux14/1 -> Angular vel/2
  Mux15/1 -> Angular vel/3
  Select 17/1 -> Mux13/1
  Select 15/1 -> Mux14/1
  Select 16/1 -> Mux15/1
  [nuBody] -> Select 17/1, Select 16/1, Select 15/1
  Demux7/2 -> attitude_estimator_q/8
  [accelero] -> attitude_estimator_q/14
  [sensor_ts] -> attitude_estimator_q/12
  [magneto_ga] -> attitude_estimator_q/16
  [nuBody] -> Gyroscope/1(nuBody)
  [gyro] -> attitude_estimator_q/13
  [q] -> Accelerometer/1(q)
  [xiDDot] -> Accelerometer/2(xiDDot)
  Accelerometer/1(accelerometer_m_s2) -> [accelero]
  Accelerometer/2(timestamp_relative) -> [accelero_tsr]
  [mocap_q] -> attitude_estimator_q/10
  [mocap_ts] -> attitude_estimator_q/11
  Gain1/1 -> Delay3/1, [timestamp]
  [timestamp] -> Mocap System/3(timestamp)
  [q] -> Mocap System/2(q)
  [xi] -> Mocap System/1(xi)
  Constant2/1 -> local_position_estimator/12
  [baro_alt] -> local_position_estimator/9
  [baro_tsr] -> local_position_estimator/10
  Mocap System/1(mocap_x) -> [mocap_x]
  Mocap System/2(mocap_y) -> [mocap_y]
  Mocap System/3(mocap_z) -> [mocap_z]
  [mocap_y] -> local_position_estimator/6
  Mocap System/4(mocap_q) -> [mocap_q]
  Mocap System/5(mocap_timestamp) -> [mocap_ts]
  attitude_estimator_q/5 -> [att_q]
  Delay3/1 -> [sensor_ts]
  [sensor_ts] -> local_position_estimator/11
  [xi] -> Barometer/1(xi)
  [timestamp] -> Barometer/2(timestamp)
  Barometer/1(baro_alt_meter) -> [baro_alt]
  Barometer/2(timestamp_relative) -> [baro_tsr]
  Gyroscope/1(gyro_rad) -> [gyro]
  [timestamp] -> Magnetometer/2(timestamp)
  Magnetometer/2(timestamp_relative) -> [magneto_tsr]
  Magnetometer/1(magnetometer_ga) -> [magneto_ga]
  [magneto_tsr] -> attitude_estimator_q/17
  Demux7/1 -> attitude_estimator_q/7
  Demux7/3 -> attitude_estimator_q/9
  [sensor_ts] -> attitude_estimator_q/6
  Mux16/1 -> [lpe_pos]
  local_position_estimator/7 -> Mux17/1
  local_position_estimator/8 -> Mux17/2
  local_position_estimator/9 -> Mux17/3
  Mux17/1 -> [lpe_vel]
  local_position_estimator/4 -> Mux18/1
  local_position_estimator/5 -> Mux18/2
  local_position_estimator/6 -> Mux18/3
  Mux18/1 -> [gpos_vel]
  local_position_estimator/1 -> [lpe_cov]
  local_position_estimator/2 -> [lpe_health]
  local_position_estimator/3 -> [lpe_states]
  [att_q] -> Quaternion to Euler Angles/1
  Mux19/1 -> Position/1
  Mux20/1 -> Position/2
  Mux21/1 -> Position/3
  Select 19/1 -> Mux21/1  "actual3"
  Select 22/1 -> Mux21/2  "est3"
  Select 21/1 -> Mux20/2  "est2"
  Select 18/1 -> Mux20/1  "actual2"
  Select 20/1 -> Mux19/2  "est1"
  Select 23/1 -> Mux19/1  "actual1"
  [lpe_pos] -> Select 20/1, Select 21/1, Select 22/1
  [lpe_cov] -> Demux5/1
  [xi] -> Select 23/1, Select 18/1, Select 19/1
  Mux1/1 -> Velocity/1
  Mux2/1 -> Velocity/2
  Mux3/1 -> Velocity/3
  Select 25/1 -> Mux3/1  "actual3"
  Select 28/1 -> Mux3/2  "est3"
  Select 27/1 -> Mux2/2  "est2"
  Select 24/1 -> Mux2/1  "actual2"
  Select 26/1 -> Mux1/2  "est1"
  Select 29/1 -> Mux1/1  "actual1"
  [lpe_vel] -> Select 28/1, Select 27/1, Select 26/1  "velEst"
  [xiDot] -> Select 25/1, Select 24/1, Select 29/1  "vel"
  Mux4/1 -> Velocity (Global)/1
  Mux5/1 -> Velocity (Global)/2
  Mux22/1 -> Velocity (Global)/3
  Select 31/1 -> Mux22/1  "actual3"
  Select 34/1 -> Mux22/2  "est3"
  Select 33/1 -> Mux5/2  "est2"
  Select 30/1 -> Mux5/1  "actual2"
  Select 32/1 -> Mux4/2  "est1"
  Select 35/1 -> Mux4/1  "actual1"
  [gpos_vel] -> Select 32/1, Select 33/1, Select 34/1
  [xiDot] -> Select 35/1, Select 30/1, Select 31/1
  [accelero] -> local_position_estimator/8
  local_position_estimator/13 -> [lpe_yaw]
  Mux/1 -> [att_nuBody]
  attitude_estimator_q/3 -> Mux/2
  attitude_estimator_q/2 -> Mux/1
  attitude_estimator_q/4 -> Mux/3
  Select 38/1 -> Mux13/2
  Select 37/1 -> Mux15/2
  [att_nuBody] -> Select 38/1, Select 36/1, Select 37/1
  Select 36/1 -> Mux14/2
  Mux23/1 -> [att_xiDDot]
  attitude_estimator_q/7 -> Mux23/2
  attitude_estimator_q/6 -> Mux23/1
  attitude_estimator_q/8 -> Mux23/3
  Mux24/1 -> Acceleration/1
  Mux25/1 -> Acceleration/2
  Mux26/1 -> Acceleration/3
  Select 41/1 -> Mux24/1  "xDDot"
  Select 39/1 -> Mux25/1  "yDDot"
  Select 40/1 -> Mux26/1  "zDDot"
  [accelero] -> Select 39/1, Select 40/1, Select 41/1
  Select 44/1 -> Mux24/2  "xDDotFilt"
  Select 43/1 -> Mux26/2  "zDDotFilt"
  [att_xiDDot] -> Select 43/1, Select 42/1, Select 44/1
  Select 42/1 -> Mux25/2  "yDDotFild"
  attitude_estimator_q/1 -> [att_timestamp]
  [att_q] -> qMeasured/1
  [gyro] -> nuBodyMeasured/1
  xiDDot/1 -> xiDDotMeasured/1, [xiDDot]
  [lpe_pos] -> xiMeasured/1
  [lpe_vel] -> xiDotMeasured/1
  Ground/1 -> attitude_estimator_q/2, attitude_estimator_q/1
  [lpe_yaw] -> Radians to Degrees2/1
  Mux27/1 -> Yaw/1
  Quaternion to Rotation Matrix/1 -> Math Function/1
  Math Function/1 -> Matrix Multiply/1
  [q] -> Quaternion to Rotation Matrix/1
  [xiDDot] -> Matrix Multiply/2
  Matrix Multiply/1 -> Select 46/1, Select 45/1, Select 50/1  "xiDDot_rot"
  [VBodyDot] -> Select 49/1, Select 48/1, Select 47/1  "VBodyDot"
  Mux31/1 -> Acc. comparison/3
  Mux29/1 -> Acc. comparison/1
  Select 46/1 -> Mux31/1  "calc3"
  Select 45/1 -> Mux30/1  "calc2"
  Select 50/1 -> Mux29/1  "calc1"
  Mux30/1 -> Acc. comparison/2
  Select 48/1 -> Mux30/2  "act2"
  Select 49/1 -> Mux31/2  "act3"
  Select 47/1 -> Mux29/2  "act1"
  Radians to Degrees/1 -> Select 11/1, Select 10/1, Select 9/1
  Radians to Degrees1/1 -> Select 14/1, Select 13/1, Select 12/1
  Radians to Degrees2/1 -> Mux27/1

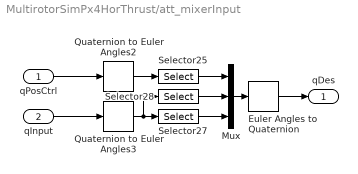
== system MultirotorSimPx4HorThrust/att_mixerInput ==
  qPosCtrl : Inport
  qInput : Inport  Port=2
  Euler Angles to Quaternion : QuaternionLibrary/Euler Angles to Quaternion
  Mux : Mux  Inputs=3
  Quaternion to Euler Angles2 : QuaternionLibrary/Quaternion to Euler Angles
  Quaternion to Euler Angles3 : QuaternionLibrary/Quaternion to Euler Angles
  Selector25 : Selector  InputPortWidth=3  IndexOptions=Index vector (dialog)  Indices=1  OutputSizes=1
  Selector27 : Selector  InputPortWidth=3  IndexOptions=Index vector (dialog)  Indices=3  OutputSizes=1
  Selector28 : Selector  InputPortWidth=3  IndexOptions=Index vector (dialog)  Indices=2  OutputSizes=1
  qDes : Outport  VectorParamsAs1DForOutWhenUnconnected=off
  wires:
  qPosCtrl/1 -> Quaternion to Euler Angles2/1
  qInput/1 -> Quaternion to Euler Angles3/1
  Euler Angles to Quaternion/1 -> qDes/1
  Mux/1 -> Euler Angles to Quaternion/1
  Quaternion to Euler Angles2/1 -> Selector25/1
  Quaternion to Euler Angles3/1 -> Selector27/1, Selector28/1
  Selector25/1 -> Mux/1
  Selector27/1 -> Mux/3
  Selector28/1 -> Mux/2

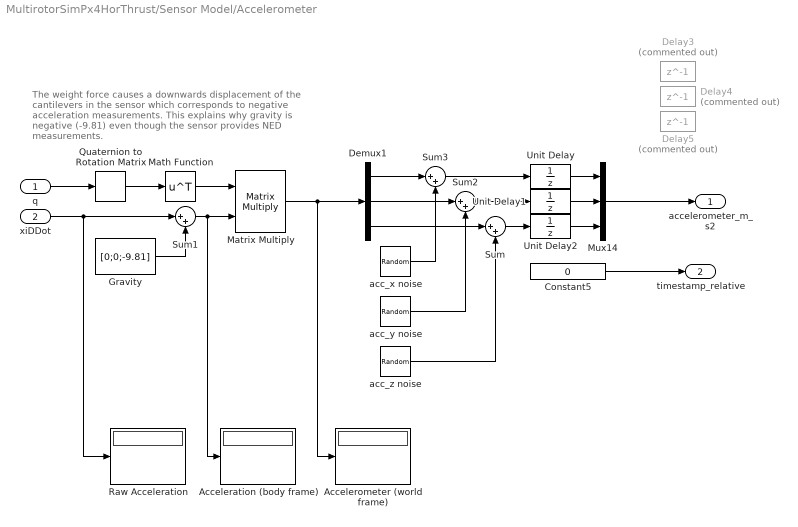
== system MultirotorSimPx4HorThrust/Sensor Model/Accelerometer ==
  note: The weight force causes a downwards displacement of
      | the cantilevers in the sensor which corresponds to
      | negative acceleration measurements. This explains why
      | gravity is negative (-9.81) even though the sensor provides
      | NED measurements.
  q : Inport
  xiDDot : Inport  Port=2  Unit=m/s^2
  Acceleration (body frame) : Display
  Accelerometer (world frame) : Display
  Constant5 : Constant  Value=0
  Delay3 : Delay  Commented=on  DelayLength=1  InitialConditionSource=Input port  SampleTime=1/400
      settings: InputPortMap=u0,p4
  Delay4 : Delay  Commented=on  DelayLength=1  InitialConditionSource=Input port  SampleTime=1/400
      settings: InputPortMap=u0,p4
  Delay5 : Delay  Commented=on  DelayLength=1  InitialConditionSource=Input port  SampleTime=1/400
      settings: InputPortMap=u0,p4
  Demux1 : Demux  Outputs=3
  Gravity : Constant  Value=[0;0;-9.81]
  Math Function : Math  Operator=transpose  SignedPower=on  SaturateOnIntegerOverflow=on
  Matrix Multiply : Product  Multiplication=Matrix(*)
  Mux14 : Mux  Inputs=3
  Quaternion to Rotation Matrix : QuaternionLibrary/Quaternion to Rotation Matrix
  Raw Acceleration : Display
  Sum{,1..3} (4 alike) : Sum  Inputs=|++
  Unit Delay : UnitDelay  SampleTime=1/400  HasFrameUpgradeWarning=on
  Unit Delay1 : UnitDelay  SampleTime=1/400  HasFrameUpgradeWarning=on
  Unit Delay2 : UnitDelay  InitialCondition=-9.81  SampleTime=1/400  HasFrameUpgradeWarning=on
  acc_x noise : RandomNumber  Variance=0.012^2  SampleTime=1/400
  acc_y noise : RandomNumber  Variance=0.012^2  SampleTime=1/400
  acc_z noise : RandomNumber  Variance=0.02^2  SampleTime=1/400
  accelerometer_m_s2 : Outport  Unit=m/s^2  SampleTime=1/400  VectorParamsAs1DForOutWhenUnconnected=off
  timestamp_relative : Outport  Port=2  Unit=µs  SampleTime=1/400  VectorParamsAs1DForOutWhenUnconnected=off
  wires:
  Quaternion to Rotation Matrix/1 -> Math Function/1
  Math Function/1 -> Matrix Multiply/1
  Matrix Multiply/1 -> Demux1/1, Accelerometer (world frame)/1
  Gravity/1 -> Sum1/2
  Sum1/1 -> Acceleration (body frame)/1, Matrix Multiply/2
  Mux14/1 -> accelerometer_m_s2/1
  q/1 -> Quaternion to Rotation Matrix/1
  Constant5/1 -> timestamp_relative/1
  Demux1/1 -> Sum3/1
  Demux1/2 -> Sum2/1
  Demux1/3 -> Sum/1
  Sum/1 -> Unit Delay2/1
  acc_z noise/1 -> Sum/2
  Sum2/1 -> Unit Delay1/1
  Sum3/1 -> Unit Delay/1
  acc_y noise/1 -> Sum2/2
  acc_x noise/1 -> Sum3/2
  Unit Delay/1 -> Mux14/1
  Unit Delay1/1 -> Mux14/2
  Unit Delay2/1 -> Mux14/3
  xiDDot/1 -> Sum1/1, Raw Acceleration/1

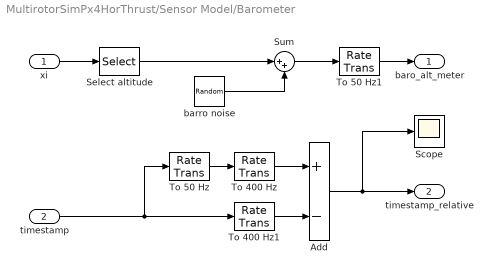
== system MultirotorSimPx4HorThrust/Sensor Model/Barometer ==
  xi : Inport  Unit=m
  timestamp : Inport  Port=2  Unit=µs
  Add : Sum  Inputs=+-
  Scope : Scope
  Select altitude : Selector  InputPortWidth=3  IndexOptions=Index vector (dialog)  Indices=3  OutputSizes=1
  Sum : Sum  Inputs=|++
  To 400 Hz : RateTransition  Deterministic=off  OutPortSampleTime=1/250
  To 400 Hz1 : RateTransition  OutPortSampleTime=1/400
  To 50 Hz : RateTransition  OutPortSampleTime=1/50
  To 50 Hz1 : RateTransition  OutPortSampleTime=1/50
  barro noise : RandomNumber  Variance=1/3^2  SampleTime=0.01
  baro_alt_meter : Outport  Unit=m  SampleTime=1/400  VectorParamsAs1DForOutWhenUnconnected=off
  timestamp_relative : Outport  Port=2  Unit=µs  VectorParamsAs1DForOutWhenUnconnected=off
  wires:
  barro noise/1 -> Sum/2
  Sum/1 -> To 50 Hz1/1
  xi/1 -> Select altitude/1
  Select altitude/1 -> Sum/1
  Add/1 -> timestamp_relative/1, Scope/1
  To 400 Hz1/1 -> Add/2
  To 50 Hz/1 -> To 400 Hz/1
  To 400 Hz/1 -> Add/1
  timestamp/1 -> To 50 Hz/1, To 400 Hz1/1
  To 50 Hz1/1 -> baro_alt_meter/1

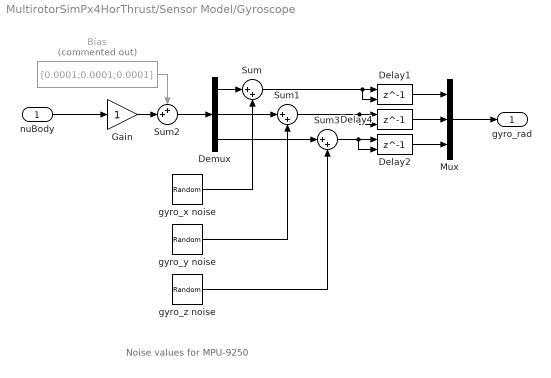
== system MultirotorSimPx4HorThrust/Sensor Model/Gyroscope ==
  note: Noise values for MPU-9250
  nuBody : Inport  Unit=rad/s
  Bias : Constant  Commented=on  Value=[0.0001;0.0001;0.0001]
  Delay1 : Delay  DelayLength=1  InitialConditionSource=Input port  SampleTime=1/400
      settings: InputPortMap=u0,p4
  Delay2 : Delay  DelayLength=1  InitialConditionSource=Input port  SampleTime=1/400
      settings: InputPortMap=u0,p4
  Delay4 : Delay  DelayLength=1  InitialConditionSource=Input port  SampleTime=1/400
      settings: InputPortMap=u0,p4
  Demux : Demux  Outputs=3
  Gain : Gain
  Mux : Mux  Inputs=3
  Sum : Sum  Inputs=|++
  Sum1 : Sum  Inputs=|++
  Sum2 : Sum  Inputs=++|
  Sum3 : Sum  Inputs=|++
  gyro_x noise : RandomNumber  Variance=(0.1*pi/180)^2  SampleTime=1/400
  gyro_y noise : RandomNumber  Variance=(0.1*pi/180)^2  SampleTime=1/400
  gyro_z noise : RandomNumber  Variance=(0.1*pi/180)^2  SampleTime=1/400
  gyro_rad : Outport  Unit=rad/s  SampleTime=1/400  VectorParamsAs1DForOutWhenUnconnected=off
  wires:
  Sum2/1 -> Demux/1
  Mux/1 -> gyro_rad/1
  Bias/1 -> Sum2/1
  nuBody/1 -> Gain/1
  Delay4/1 -> Mux/2
  Delay2/1 -> Mux/3
  Delay1/1 -> Mux/1
  Sum/1 -> Delay1/2, Delay1/1
  Sum1/1 -> Delay4/2, Delay4/1
  Sum3/1 -> Delay2/2, Delay2/1
  Gain/1 -> Sum2/2
  Demux/1 -> Sum/1
  Demux/2 -> Sum1/1
  Demux/3 -> Sum3/1
  gyro_x noise/1 -> Sum/2
  gyro_y noise/1 -> Sum1/2
  gyro_z noise/1 -> Sum3/2

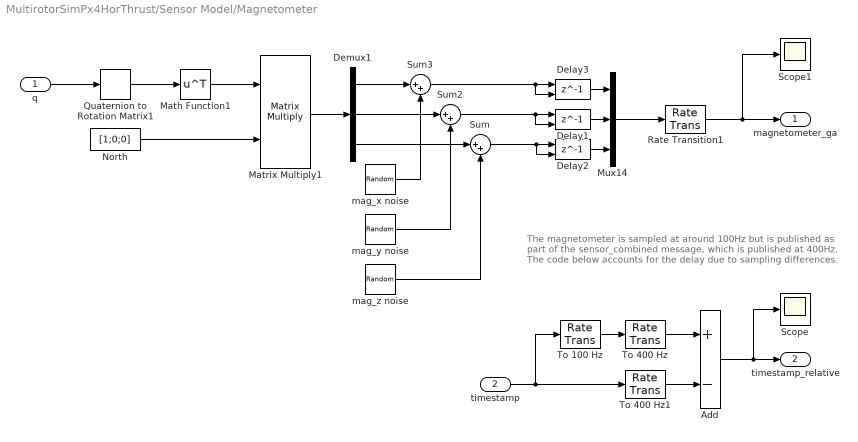
== system MultirotorSimPx4HorThrust/Sensor Model/Magnetometer ==
  note: The magnetometer is sampled at around 100Hz but is published
      | as part of the sensor_combined message, which is published at
      | 400Hz. The code below accounts for the delay due to sampling
      | differences.
  q : Inport
  timestamp : Inport  Port=2
  Add : Sum  Inputs=+-
  Delay1 : Delay  DelayLength=1  InitialConditionSource=Input port  SampleTime=1/100
      settings: InputPortMap=u0,p4
  Delay2 : Delay  DelayLength=1  InitialConditionSource=Input port  SampleTime=1/100
      settings: InputPortMap=u0,p4
  Delay3 : Delay  DelayLength=1  InitialConditionSource=Input port  SampleTime=1/100
      settings: InputPortMap=u0,p4
  Demux1 : Demux  Outputs=3
  Math Function1 : Math  Operator=transpose  SignedPower=on  SaturateOnIntegerOverflow=on
  Matrix Multiply1 : Product  Multiplication=Matrix(*)
  Mux14 : Mux  Inputs=3
  North : Constant  Value=[1;0;0]
  Quaternion to Rotation Matrix1 : QuaternionLibrary/Quaternion to Rotation Matrix
  Rate Transition1 : RateTransition  Deterministic=off  OutPortSampleTime=1/100
  Scope : Scope
  Scope1 : Scope
  Sum : Sum  Inputs=|++
  Sum2 : Sum  Inputs=|++
  Sum3 : Sum  Inputs=|++
  To 100 Hz : RateTransition  OutPortSampleTime=1/100
  To 400 Hz : RateTransition  Deterministic=off  OutPortSampleTime=1/250
  To 400 Hz1 : RateTransition  OutPortSampleTime=1/400
  mag_x noise : RandomNumber  Variance=0.001^2  SampleTime=1/400
  mag_y noise : RandomNumber  Variance=0.001^2  SampleTime=1/400
  mag_z noise : RandomNumber  Variance=0.001^2  SampleTime=1/400
  magnetometer_ga : Outport  Unit=G  SampleTime=1/250  VectorParamsAs1DForOutWhenUnconnected=off
  timestamp_relative : Outport  Port=2  Unit=µs  SampleTime=1/250  VectorParamsAs1DForOutWhenUnconnected=off
  wires:
  q/1 -> Quaternion to Rotation Matrix1/1
  Quaternion to Rotation Matrix1/1 -> Math Function1/1
  North/1 -> Matrix Multiply1/2
  Math Function1/1 -> Matrix Multiply1/1
  Add/1 -> timestamp_relative/1, Scope/1
  Matrix Multiply1/1 -> Demux1/1
  Demux1/1 -> Sum3/1
  Demux1/2 -> Sum2/1
  Demux1/3 -> Sum/1
  Sum/1 -> Delay2/2, Delay2/1
  mag_z noise/1 -> Sum/2
  Sum2/1 -> Delay1/2, Delay1/1
  mag_y noise/1 -> Sum2/2
  mag_x noise/1 -> Sum3/2
  Mux14/1 -> Rate Transition1/1
  To 400 Hz1/1 -> Add/2
  To 100 Hz/1 -> To 400 Hz/1
  To 400 Hz/1 -> Add/1
  Rate Transition1/1 -> Scope1/1, magnetometer_ga/1
  timestamp/1 -> To 100 Hz/1, To 400 Hz1/1
  Delay3/1 -> Mux14/1
  Sum3/1 -> Delay3/2, Delay3/1
  Delay1/1 -> Mux14/2
  Delay2/1 -> Mux14/3
